simulink model "Sim_2"  (R2016a)
settings: Solver=VariableStepAuto  StartTime=0.0  StopTime=500  RelTol=1e-3
undefined symbols (not defined in the file or in its folder): des, gcbh
settings Model: Creator=Lenovo  LastModifiedBy=Lenovo

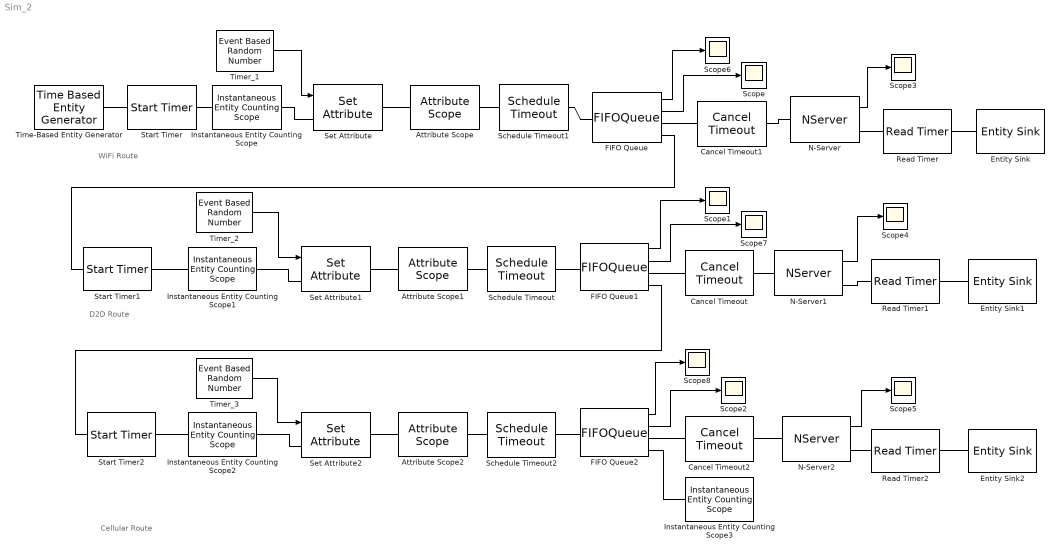
== system Sim_2 ==
  note: Cellular Route
  note: D2D Route
  note: WiFi Route
  Attribute Scope : AttributeScope  LoadFcn=des.scope.CallbackSupport('seLoadFcn',gcbh)  StartFcn=des.scope.CallbackSupport('seStartFcn',gcbh)  StopFcn=des.scope.CallbackSupport('seStopFcn',gcbh)  AttributeNameY=Timer  Title=X Value from Event Time  XLabel=Event Time (s)  YLabel=No. of Entities in Queue
      settings: CopyFcn=des.scope.CallbackSupport('seCopyFcn',gcbh)  DeleteFcn=des.scope.CallbackSupport('seDeleteFcn',gcbh)  PreSaveFcn=des.scope.CallbackSupport('sePreSaveFcn',gcbh)  NameChangeFcn=des.scope.CallbackSupport('seNameChangeFcn',gcbh)  OpenFcn=des.scope.CallbackSupport('seOpenFcn',gcbh)
  Attribute Scope1 : AttributeScope  LoadFcn=des.scope.CallbackSupport('seLoadFcn',gcbh)  StartFcn=des.scope.CallbackSupport('seStartFcn',gcbh)  StopFcn=des.scope.CallbackSupport('seStopFcn',gcbh)  AttributeNameY=Timer_2  Title=X Value from Event Time  XLabel=Event Time (s)  YLabel=No. of Entities in Queue
      settings: CopyFcn=des.scope.CallbackSupport('seCopyFcn',gcbh)  DeleteFcn=des.scope.CallbackSupport('seDeleteFcn',gcbh)  PreSaveFcn=des.scope.CallbackSupport('sePreSaveFcn',gcbh)  NameChangeFcn=des.scope.CallbackSupport('seNameChangeFcn',gcbh)  OpenFcn=des.scope.CallbackSupport('seOpenFcn',gcbh)
  Attribute Scope2 : AttributeScope  LoadFcn=des.scope.CallbackSupport('seLoadFcn',gcbh)  StartFcn=des.scope.CallbackSupport('seStartFcn',gcbh)  StopFcn=des.scope.CallbackSupport('seStopFcn',gcbh)  AttributeNameY=Timer_3  Title=X Value from Event Time  XLabel=Event Time (s)  YLabel=No. of Entities in Queue
      settings: CopyFcn=des.scope.CallbackSupport('seCopyFcn',gcbh)  DeleteFcn=des.scope.CallbackSupport('seDeleteFcn',gcbh)  PreSaveFcn=des.scope.CallbackSupport('sePreSaveFcn',gcbh)  NameChangeFcn=des.scope.CallbackSupport('seNameChangeFcn',gcbh)  OpenFcn=des.scope.CallbackSupport('seOpenFcn',gcbh)
  Cancel Timeout : CancelTimeout  TimeoutTag=TO2
  Cancel Timeout1 : CancelTimeout
  Cancel Timeout2 : CancelTimeout  TimeoutTag=TO3
  Entity Sink : EntitySink
  Entity Sink1 : EntitySink
  Entity Sink2 : EntitySink
  FIFO Queue : FIFOQueue  Capacity=Inf  EnableTOPort=on  StatNumberInBlock=on  StatAverageQueueLength=on
      settings: OutputPortMap=o1,o3
  FIFO Queue1 : FIFOQueue  Capacity=Inf  EnableTOPort=on  StatNumberInBlock=on  StatAverageQueueLength=on
      settings: OutputPortMap=o1,o3
  FIFO Queue2 : FIFOQueue  Capacity=Inf  EnableTOPort=on  StatNumberInBlock=on  StatAverageQueueLength=on
      settings: OutputPortMap=o1,o3
  Instantaneous Entity Counting Scope{,1..3} (4 alike) : InstantaneousEntityCountingScope  LoadFcn=des.scope.CallbackSupport('seLoadFcn',gcbh)  StartFcn=des.scope.CallbackSupport('seStartFcn',gcbh)  StopFcn=des.scope.CallbackSupport('seStopFcn',gcbh)
      settings: CopyFcn=des.scope.CallbackSupport('seCopyFcn',gcbh)  DeleteFcn=des.scope.CallbackSupport('seDeleteFcn',gcbh)  PreSaveFcn=des.scope.CallbackSupport('sePreSaveFcn',gcbh)  NameChangeFcn=des.scope.CallbackSupport('seNameChangeFcn',gcbh)  OpenFcn=des.scope.CallbackSupport('seOpenFcn',gcbh)
  N-Server : NServer  NumberOfServers=1  ServiceTimeFrom=Attribute  AttributeName=Patience  StatUtilization=on
      settings: OutputPortMap=o5
  N-Server1 : NServer  NumberOfServers=1  ServiceTimeFrom=Attribute  AttributeName=Patience  StatUtilization=on
      settings: OutputPortMap=o5
  N-Server2 : NServer  NumberOfServers=1  ServiceTimeFrom=Attribute  AttributeName=Patience  StatUtilization=on
      settings: OutputPortMap=o5
  Read Timer : ReadTimer
  Read Timer1 : ReadTimer
  Read Timer2 : ReadTimer
  Schedule Timeout : ScheduleTimeout  TimeoutTag=TO2  TimeoutIntervalFrom=Attribute  AttributeName=Timer_2
  Schedule Timeout1 : ScheduleTimeout  TimeoutIntervalFrom=Attribute  AttributeName=Timer
  Schedule Timeout2 : ScheduleTimeout  TimeoutTag=TO3  TimeoutIntervalFrom=Attribute  AttributeName=Timer_3
  Scope{,1..8} (9 alike) : Scope
  Set Attribute : SetAttribute  AttributeName=Timer|Patience  AttributeFrom=Signal port|Dialog  AttributeValue=1|1  AttributeTreatAsVector=1|1  EvaluatedAttributeValue={ [];1}
  Set Attribute1 : SetAttribute  AttributeName=Timer_2|Patience  AttributeFrom=Signal port|Dialog  AttributeValue=1|1  AttributeTreatAsVector=1|1  EvaluatedAttributeValue={ [];1}
  Set Attribute2 : SetAttribute  AttributeName=Timer_3|Patience  AttributeFrom=Signal port|Dialog  AttributeValue=1|1  AttributeTreatAsVector=1|1  EvaluatedAttributeValue={ [];1}
  Start Timer : StartTimer
  Start Timer1 : StartTimer
  Start Timer2 : StartTimer
  Time-Based Entity Generator : TimeBasedEntityGenerator  Distribution=Exponential  InitialSeed=30384  Mean=1/60
  Timer_1 : EventBasedRandomNumber  Distribution=Poisson  maxUnif=120  meanNorm=90  stdNorm=80  meanPoiss=120  Seed=3452
  Timer_2 : EventBasedRandomNumber  Distribution=Poisson  minUnif=10  maxUnif=500  meanNorm=90  stdNorm=80  meanPoiss=30  Seed=12346
  Timer_3 : EventBasedRandomNumber  Distribution=Poisson  minUnif=10  maxUnif=500  meanNorm=90  stdNorm=80  meanPoiss=120  Seed=12347
  wires:
  Timer_1/1 -> Set Attribute/1
  Timer_2/1 -> Set Attribute1/1
  Timer_3/1 -> Set Attribute2/1
  FIFO Queue/2 -> Scope/1
  N-Server/1 -> Scope3/1
  N-Server1/1 -> Scope4/1
  N-Server2/1 -> Scope5/1
  FIFO Queue/1 -> Scope6/1
  FIFO Queue1/1 -> Scope1/1
  FIFO Queue1/2 -> Scope7/1
  FIFO Queue2/2 -> Scope2/1
  FIFO Queue2/1 -> Scope8/1
  connections:
  FIFO Queue/LConn1 -- Schedule Timeout1/RConn1
  Start Timer/LConn1 -- Time-Based Entity Generator/RConn1
  Set Attribute/LConn1 -- Instantaneous Entity Counting Scope/RConn1
  Cancel Timeout1/LConn1 -- FIFO Queue/RConn1
  Read Timer/LConn1 -- N-Server/RConn1
  Attribute Scope1/LConn1 -- Set Attribute1/RConn1
  Set Attribute1/LConn1 -- Instantaneous Entity Counting Scope1/RConn1
  Read Timer1/LConn1 -- N-Server1/RConn1
  Cancel Timeout/LConn1 -- FIFO Queue1/RConn1
  Schedule Timeout/LConn1 -- Attribute Scope1/RConn1
  FIFO Queue1/LConn1 -- Schedule Timeout/RConn1
  N-Server1/LConn1 -- Cancel Timeout/RConn1
  Schedule Timeout1/LConn1 -- Attribute Scope/RConn1
  N-Server/LConn1 -- Cancel Timeout1/RConn1
  FIFO Queue/RConn2 -- Start Timer1/LConn1
  FIFO Queue2/LConn1 -- Schedule Timeout2/RConn1
  Cancel Timeout2/LConn1 -- FIFO Queue2/RConn1
  Set Attribute2/LConn1 -- Instantaneous Entity Counting Scope2/RConn1
  Schedule Timeout2/LConn1 -- Attribute Scope2/RConn1
  Read Timer2/LConn1 -- N-Server2/RConn1
  Attribute Scope2/LConn1 -- Set Attribute2/RConn1
  N-Server2/LConn1 -- Cancel Timeout2/RConn1
  FIFO Queue1/RConn2 -- Start Timer2/LConn1
  FIFO Queue2/RConn2 -- Instantaneous Entity Counting Scope3/LConn1
  Attribute Scope/LConn1 -- Set Attribute/RConn1
  Instantaneous Entity Counting Scope/LConn1 -- Start Timer/RConn1
  Entity Sink/LConn1 -- Read Timer/RConn1
  Entity Sink1/LConn1 -- Read Timer1/RConn1
  Entity Sink2/LConn1 -- Read Timer2/RConn1
  Start Timer1/RConn1 -- Instantaneous Entity Counting Scope1/LConn1
  Start Timer2/RConn1 -- Instantaneous Entity Counting Scope2/LConn1
